simulink model "Subsystem1"  (R2020b)
settings: Solver=VariableStepAuto  StartTime=0.0  StopTime=10.0  RelTol=1e-3
undefined symbols (not defined in the file): Ki, Kp
settings Model: Creator=Pulkit Khandelwal  LastModifiedBy=Pulkit Khandelwal
settings DataIOCC: SaveOutput=off  SaveTime=off

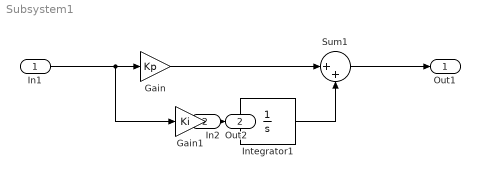
== system Subsystem1 ==
  In1 : Inport  OutDataTypeStr=double  PortDimensions=1  SampleTime=0
  In2 : Inport  Port=2  OutDataTypeStr=double  PortDimensions=1
  Gain : Gain  Gain=Kp
  Gain1 : Gain  Gain=Ki
  Integrator1 : Integrator
  Sum1 : Sum  Inputs=|++
  Out1 : Outport  OutDataTypeStr=double  PortDimensions=1  SampleTime=0
  Out2 : Outport  Port=2  OutDataTypeStr=double  PortDimensions=1  SampleTime=0
  wires:
  Sum1/1 -> Out1/1
  Integrator1/1 -> Sum1/2
  Gain/1 -> Sum1/1
  In1/1 -> Gain1/1, Gain/1
  In2/1 -> Integrator1/1
  Gain1/1 -> Out2/1
